simulink model "mvmama001_stltse004"  (R2021a)
settings: Solver=FixedStepAuto  StartTime=0.0  StopTime=500  RelTol=1e-3
undefined symbols (not defined in the file or in its folder): InputPWM, WheelSpeed
libraries: arduinolib x10, pid_lib x1, mobileRoboticsTrainingLib x1
settings Model: SILPILModeSetting=veronly  ExtModeTrigDuration=2  Creator=User  LastModifiedBy=Amandla Mvimbi
settings OptimizationCC: EnhancedBackFolding=on  PassReuseOutputArgsAs=Individual arguments  ZeroExternalMemoryAtStartup=off  ZeroInternalMemoryAtStartup=off  MaxStackSize=64  OptimizeBlockOrder=speed  DifferentSizesBufferReuse=on  EfficientTunableParamExpr=on
settings DebuggingCC: ParameterTunabilityLossMsg=error
settings HardwareCC: ProdBitPerInt=16  ProdBitPerPointer=16  ProdBitPerSizeT=16  ProdBitPerPtrDiffT=16  ProdLargestAtomicFloat=None  ProdWordSize=8  ProdHWDeviceType=Atmel->AVR  UseEmbeddedCoderFeatures=off  UseSimulinkCoderFeatures=off
settings SFSimCC: MATLABDynamicMemAlloc=off
settings RTWCC: SystemTargetFile=ert.tlc  HardwareBoard=Arduino Leonardo  TemplateMakefile=ert_default_tmf  Toolchain=Arduino AVR
settings CodeAppCC: ForceParamTrailComments=on  IgnoreCustomStorageClasses=off  OperatorAnnotations=on  SimulinkDataObjDesc=on  SFDataObjDesc=on  InsertBlockDesc=on
settings ERTTargetCC: SupportContinuousTime=on  SupportNonInlinedSFcns=on  SupportVariableSizeSignals=on  ExtModeTransport=5  ExtModeStaticAllocSize=250  ExtModeMexFile=ext_serial_win32_comm_leonardo

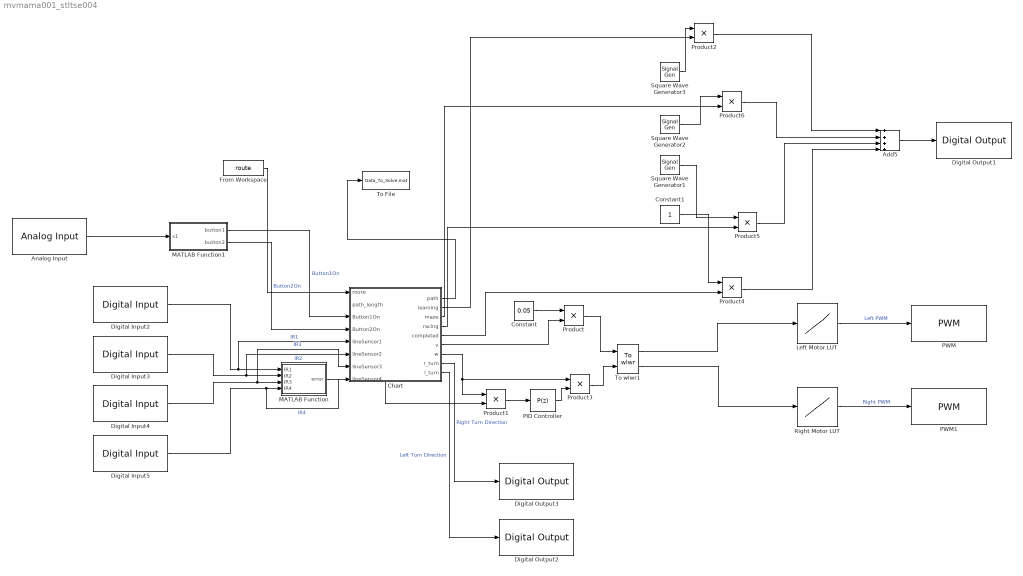
== system mvmama001_stltse004 ==
  Add5 : Sum  Inputs=++++
  Analog Input : arduinolib/Analog Input  pinNumber=0  ReadResultsOnly=off  ConversionTriggerSource=Software  ExternalTriggerType=uint32( 0 )  OutputDataType=uint16  EnableConversionCompleteNotify=off  EnableOuputStatus=off  SampleTime=-1  blockPlatform=arduino
  Chart : Stateflow chart  TreatAsAtomicUnit=on
      settings: PortSchema="{\"entries\":[{\"content\":{\"sides\":[{\"content\":{\"connectorIds\":[\"In7\",\"In8\",\"In1\",\"In2\",\"In3\",\"In5\",\"In4\",\"In6\"]},\"type\":\"ConnectorPlacement.EquallySpacedRectSide\",\"uuid\":\"badfc6b2-29c2-4b15-bfb9-62e4da121403\"},{\"content\":{\"connectorIds\":[\"Out9\",\"Out1\",\"Out3\",\"Out4\",\"Out2\",\"Out5\",\"Out6\",\"Out8\",\"Out7\"],\"side\":\"RIGHT\"},\"type\":\"ConnectorPlacement.EquallySpacedRectSide\",\"uuid\":\"19ffdcd3-74e5-47dc-b9d4-6ea0e9598c3b\"},{\"content\":{\"connectorIds\":[],\"side\":\"TOP\"},\"type\":\"ConnectorPlacement.EquallySpacedRectSide\",\"uuid\":\"4f1e845d-b34d-4676-ae53-c7ee998e6419\"}]},\"type\":\"ConnectorPlacement.EquallySpacedConnector\",\"uuid\":\"d87d8507-4bd7-4ce8-9c9b-ea7230bf73eb\"}],\"packageUris\":[\"http://schema.mathworks.com/mf0/Connector/R2020b\"],\"version\":\"1.0\"}"
  Constant : Constant  Value=0.05
  Constant1 : Constant
  Digital Input2 : arduinolib/Digital Input  pinNumber=8  mode=Default  Direction=input  SampleTime=0.1  blockPlatform=arduino
  Digital Input3 : arduinolib/Digital Input  pinNumber=9  mode=Default  Direction=input  SampleTime=0.1  blockPlatform=arduino
  Digital Input4 : arduinolib/Digital Input  pinNumber=10  mode=Default  Direction=input  SampleTime=0.1  blockPlatform=arduino
  Digital Input5 : arduinolib/Digital Input  pinNumber=11  mode=Default  Direction=input  SampleTime=0.1  blockPlatform=arduino
  Digital Output1 : arduinolib/Digital Output  pinNumber=13  Direction=output  blockPlatform=arduino
  Digital Output2 : arduinolib/Digital Output  pinNumber=4  Direction=output  blockPlatform=arduino
  Digital Output3 : arduinolib/Digital Output  pinNumber=7  Direction=output  blockPlatform=arduino
  From Workspace : FromWorkspace  VariableName=route
  Left Motor LUT : Lookup_n-D  NumberOfTableDimensions=1  BreakpointsForDimension1=WheelSpeed  Table=InputPWM  InterpMethod=Nearest  ExtrapMethod=Clip  InternalRulePriority=Speed  RndMeth=Simplest  InputSameDT=on
  MATLAB Function : MATLAB Function  TreatAsAtomicUnit=on
  MATLAB Function1 : MATLAB Function  TreatAsAtomicUnit=on
  PID Controller : pid_lib/PID Controller  Controller=P  Form=Parallel  TimeDomain=Discrete-time  UseExternalTs=off  SampleTime=-1  IntegratorMethod=Forward Euler  FilterMethod=Forward Euler  ControllerParametersSource=internal  P=0.6  I=0.8  D=1e-8  UseFilter=on  N=100  TunerSelectOption=Transfer Function Based (PID Tuner App)  InitialConditionSource=internal  InitialConditionForIntegrator=2  InitialConditionForFilter=0  DifferentiatorICPrevScaledInput=0  ExternalReset=none  TrackingMode=off  Kt=1  LimitOutput=off  SatLimitsSource=internal  UpperSaturationLimit=inf  LowerSaturationLimit=-inf  LinearizeAsGain=on  AntiWindupMode=none  Kb=1  POutMin=[]  POutMax=[]  IOutMin=[]  IOutMax=[]  DOutMin=[]  DOutMax=[]  NOutMin=[]  NOutMax=[]  SumOutMin=[]  SumOutMax=[]  SaturationOutMin=[]  SaturationOutMax=[]  PParamMin=[]  PParamMax=[]  IParamMin=[]  IParamMax=[]  DParamMin=[]  DParamMax=[]  NParamMin=[]  NParamMax=[]  KbParamMin=[]  KbParamMax=[]  KtParamMin=[]  KtParamMax=[]  KbOutMin=[]  KbOutMax=[]  KtOutMin=[]  KtOutMax=[]  IntegratorOutMin=[]  IntegratorOutMax=[]  FilterOutMin=[]  FilterOutMax=[]  SumI1OutMin=[]  SumI1OutMax=[]  SumI2OutMin=[]  SumI2OutMax=[]  SumI3OutMin=[]  SumI3OutMax=[]  SumI4OutMin=[]  SumI4OutMax=[]  SumDOutMin=[]  SumDOutMax=[]  DifferentiatorOutMin=[]  DifferentiatorOutMax=[]  FilterDiffOutCoefMin=[]  FilterDiffOutCoefMax=[]  ReciprocalOutMin=[]  ReciprocalOutMax=[]  SumDenOutMin=[]  SumDenOutMax=[]  SumNumOutMin=[]  SumNumOutMax=[]  DivideOutMin=[]  DivideOutMax=[]  UdiffTsProdOutMin=[]  UdiffTsProdOutMax=[]  NTsProdOutMin=[]  NTsProdOutMax=[]  UintegralTsProdOutMin=[]  UintegralTsProdOutMax=[]  UngainTsProdOutMin=[]  UngainTsProdOutMax=[]  IntegratorContinuousStateAttributes=''  IntegratorStateMustResolveToSignalObject=off  IntegratorRTWStateStorageClass=Auto  FilterContinuousStateAttributes=''  FilterStateMustResolveToSignalObject=off  FilterRTWStateStorageClass=Auto  ParallelPVariant=InternalParameters  IdealPVariant=Disabled  IVariant=Disabled  DVariant=Disabled  IntegratorVariant=Disabled  SatVariant=Disabled  AWVariant=Disabled  PCopyVariant=Disabled  TRVariant=Disabled  FdbkBlocksVariant=Forward  IdealPFdbkVariant=Disabled  SatFdbkVariant=Disabled  DerivativeFilterVariant=Disabled  NVariant=Disabled  NCopyVariant=Disabled_SignalSpec  FilterICVariant=Disabled  IntegratorICVariant=Disabled  ExternalResetVariant=Disabled  TRSumVariant=Passthrough  SumFdbkVariant=Disabled  SumVariant=Passthrough_P  TsampFilterVariant=InternalTs  TsampNgainVariant=Passthrough  TsampIntegralVariant=Disabled_SignalSpec  ExternalSaturationOutDataTypeStr=Inherit: Same as second input
  PWM : arduinolib/PWM  pinNumber=5  frequencyType=Default  desiredFrequency=490.2  achievableFrequency=490.2
  PWM1 : arduinolib/PWM  pinNumber=6  frequencyType=Default  desiredFrequency=490.2  achievableFrequency=490.2
  Product{,1..6} (7 alike) : Product
  Right Motor LUT : Lookup_n-D  NumberOfTableDimensions=1  BreakpointsForDimension1=WheelSpeed  Table=InputPWM  InterpMethod=Nearest  ExtrapMethod=Clip  InternalRulePriority=Speed  RndMeth=Simplest  InputSameDT=on
  Square Wave Generator1 : SignalGenerator  WaveForm=square  Frequency=5
  Square Wave Generator2 : SignalGenerator  WaveForm=square  Frequency=2
  Square Wave Generator3 : SignalGenerator  WaveForm=square
  To File : ToFile  Filename=Data_To_Solve.mat  MatrixName=path_raw  SampleTime=5
  To wlwr1 : mobileRoboticsTrainingLib/To wlwr  axleLength=axleLength  wheelR=wheelR
  wires:
  Product1/1 -> PID Controller/1
  MATLAB Function/1(error) -> Product1/2
  Product/1 -> To wlwr1/1
  Right Motor LUT/1 -> PWM1/1  "Right PWM"
  Square Wave Generator1/1 -> Product5/1
  Add5/1 -> Digital Output1/1
  Chart/4(racing) -> Product5/2
  Chart/2(completed) -> Product4/2
  Square Wave Generator2/1 -> Product6/1
  Constant/1 -> Product/1
  MATLAB Function1/1(button1) -> Chart/1(Button1On)  "Button1On"
  Product4/1 -> Add5/4
  Product6/1 -> Add5/2
  Constant1/1 -> Product4/1
  Product5/1 -> Add5/3
  Digital Input3/1 -> Chart/5(lineSensor2), MATLAB Function/2(IR2)  "IR2"
  Digital Input2/1 -> Chart/3(lineSensor1), MATLAB Function/1(IR1)  "IR1"
  Chart/3(maze) -> Product6/2
  Chart/6(w) -> Product1/1, Product3/1
  Digital Input4/1 -> Chart/4(lineSensor3), MATLAB Function/3(IR3)  "IR3"
  Analog Input/1 -> MATLAB Function1/1(s1)
  Left Motor LUT/1 -> PWM/1  "Left PWM"
  Digital Input5/1 -> Chart/6(lineSensor4), MATLAB Function/4(IR4)  "IR4"
  Product3/1 -> To wlwr1/2
  Chart/8(r_turn) -> Digital Output3/1  "Right Turn Direction"
  Square Wave Generator3/1 -> Product2/1
  Product2/1 -> Add5/1
  Chart/1(learning) -> Product2/2
  MATLAB Function1/2(button2) -> Chart/2(Button2On)  "Button2On"
  Chart/5(v) -> Product/2
  PID Controller/1 -> Product3/2
  To wlwr1/2 -> Right Motor LUT/1
  To wlwr1/1 -> Left Motor LUT/1
  Chart/7(l_turn) -> Digital Output2/1  "Left Turn Direction"
  Chart/9(path) -> To File/1
  From Workspace/1 -> Chart/7(route)

== matlab function mvmama001_stltse004/MATLAB Function1 ==
  data: s1 input; button1 output; button2 output
function [button1, button2] = fcn(s1)
p1 = 0;
p2 = 0;
if s1 <= 100
    p1 = 1;
end
if s1 > 100 && s1 < 200
    p2 = 1;
end
button1 = p1;
button2 = p2;

== matlab function mvmama001_stltse004/MATLAB Function ==
  data: IR1 input; error output; IR2 input; IR3 input; IR4 input
function error = fcn(IR1, IR2, IR3, IR4)
% Sets the number of sensors on the line to 0
numberof0 = 0;
% Checks if IR2 is on the line
if IR2 == 0 
    % Increments the count of number of sensors on the line
    numberof0 = numberof0 + 1; 
end
% Checks if IR3 is on the line
if IR3 == 0 
    % Increments the count of number of sensors on the line
    numberof0 = numberof0 + 1; 
end
% If neither of the two middle sensors are on the line, stop the robot
if numberof0 == 0 
    CurrentDeveation = 0;
else
    % This formula determines the currevnt deviation of the robot
    CurrentDeveation = ((IR2*2)+(IR3*-2))/numberof0;
end
% Calculates the error from the current deviation
error = 0 - CurrentDeveation;

== stateflow chart mvmama001_stltse004/Chart ==
  state RightT1
    entry:
    v=1;
    w=1;
    r_turn=-1;
    l_turn =-1;
    length1=length1+1;
  state Button1_On
    entry:
    learning =1;
    v=-1;
    w=-1;
    r_turn=-1;
    l_turn=-1;
    length1=1;
    path = zeros(1,100);
  state Start
    entry:
    completed = 0;
    maze=0;
    learning =0;
    racing =0;
    v=0;
    w=0;
    r_turn=-1;
    l_turn=-1;
    length1=0;
    path = zeros(1,100);
  state Junction_Detect
    entry:
    v=1;
    length1=length1+1;
  state Forward
    entry:
    v=1;
  state Button2_On
    entry:
    direction= 0;
    v=-1;
    w=-1;
    r_turn=-1;
    l_turn=-1;
    length1= 2;
    maze= 0;
    racing =1;
  state Right
    entry:
    v=0;
  state Junction_Detect1
    entry:
    v=1;
    direction = route(path_length+1);
  state Forward1
    entry:
    v=1;
  state Right1
    entry:
    v=0;
  state Left
    entry:
    v=0;
  state Straight
    entry:
    v=1;
  state Cross
  state Left1
    entry:
    v=0;
  state Straight1
    entry:
    v=1;
  state Right_Detect
    entry:
    v=1;
    w=0;
    r_turn=1;
    l_turn =-1;
  state Cross1
  state Backward
    entry:
    v=1;
    w=1;
    r_turn=-1;
    l_turn =-1;
    path(length1)=2;
  state Check
    entry:
    v=-0.5;
  state Check2
  state Right_Detect1
    entry:
    v=1;
    w=0;
    r_turn=1;
    l_turn =-1;
  state Straight_Detect
    entry:
    v=0;
  state Left_Detect
    entry:
    v=1;
    w=0;
    r_turn=-1;
    l_turn =1;
  state Check3
    entry:
    v=-0.5;
  state Check4
  state Stop1
    entry:
    completed=1;
    racing =1;
    v=0;
    w=0;
    r_turn=-1;
    l_turn =-1;
  state Straight_Detect1
    entry:
    l_turn=1;
    r_turn =-1;
    v=1;
  state Left_Detect1
    entry:
    v=1;
    w=0;
    r_turn=-1;
    l_turn =1;
  state RightTurn
    entry:
    v=1;
    w=0;
    r_turn=1;
    l_turn =-1;
  state RightT
    entry:
    v=1;
    w=1;
    r_turn=-1;
    l_turn =-1;
    path(length1)=4;
  state Continue
    entry:
    v=1;
    w=1;
    r_turn=-1;
    l_turn =-1;
    path(length1)=3;
  state RightTurn1
    entry:
    v=1;
    w=0;
    r_turn=1;
    l_turn =-1;
  state LeftT
    entry:
    v=0;
    w=1;
    r_turn=-1;
    l_turn =-1;
    path(length1)=1;
  state Continue1
    entry:
    v=1;
    w=1;
    r_turn=-1;
    l_turn =-1;
    length1=length1+1;
  state LeftTurn
    entry:
    v=1;
    w=0;
    r_turn=-1;
    l_turn =1;
  state LeftT1
    entry:
    v=0;
    w=1;
    r_turn=-1;
    l_turn =-1;
    length1=length1+1;
  state LeftTurn1
    entry:
    v=1;
    w=0;
    r_turn=-1;
    l_turn =1;
  state DeadEnd
    entry:
    v=1;
    w=0;
    r_turn=-1;
    l_turn =1;
  state DeadEnd1
    entry:
    v=1;
    w=0;
    r_turn=-1;
    l_turn =1;
  state TurnAround
    entry:
    v=1;
    w=0;
    r_turn=-1;
    l_turn =1;
  state Backward1
    entry:
    v=1;
    w=1;
    r_turn=-1;
    l_turn =-1;
    path(length1)=2;
  state TurnAround1
    entry:
    v=1;
    w=0;
    r_turn=-1;
    l_turn =1;
  state Stop
    entry:
    learning =0;
    maze =1;
    v=0;
    w=0;
    r_turn=-1;
    l_turn =-1;
  state crossVerification
    entry:
    v = 1;
  RightT -> Forward
  Continue -> Forward
  RightT1 -> Forward1
  Continue1 -> Forward1
  (default) -> Start
  RightTurn1 -> RightT1 : [lineSensor2==0&&lineSensor3==0]
  Button1_On -> Forward
  Forward -> Junction_Detect : [lineSensor1 == 0 || lineSensor2 == 1&& lineSensor3 == 1|| lineSensor4 == 0 ]
  Junction_Detect -> Right [order 1] : [lineSensor4 ==0&&lineSensor1~=0]
  Backward -> Forward
  Start -> Button1_On : [Button1On==1]
  LeftT -> Forward
  Right -> Continue [order 2] : after(1,sec)
  Junction_Detect -> Left [order 3] : [lineSensor1==0]
  Junction_Detect -> Straight [order 2] : after(0.6,sec)[lineSensor2==1&&lineSensor3==1]
  Button2_On -> Forward1
  Forward1 -> Junction_Detect1 : [lineSensor1 == 0 || lineSensor2 == 1&& lineSensor3 == 1|| lineSensor4 == 0 ]
  Junction_Detect1 -> Right1 [order 1] : [direction ==4]
  Right -> Right_Detect [order 1] : [lineSensor4 ==0 && lineSensor2 ==1&& lineSensor3==1]
  Backward1 -> Forward1
  LeftT1 -> Forward1
  Junction_Detect1 -> Left1 [order 3] : [direction==1]
  Junction_Detect1 -> Straight1 [order 2] : [direction ==3]
  Junction_Detect1 -> Stop1 [order 4] : [direction ==0]
  Right1 -> Continue1 [order 1] : after(1,sec)
  Right1 -> Right_Detect1 [order 2] : [lineSensor4 ==0 && lineSensor2 ==1&& lineSensor3==1]
  Stop -> Button2_On : [Button2On == 1]
  Left -> Cross [order 2] : [lineSensor1==0&&lineSensor2==0&&lineSensor3==0&&lineSensor4==0]
  Left -> Check [order 1] : [lineSensor1==0&&lineSensor2==1&&lineSensor3==1]
  Cross -> Check2 : after(1,sec)
  Left -> Left_Detect [order 3] : after(1,sec)
  Straight -> Straight_Detect : after(0.2,sec)
  Left1 -> Cross1 [order 2] : [lineSensor1==0&&lineSensor2==0&&lineSensor3==0&&lineSensor4==0]
  Left1 -> Check3 [order 1] : [lineSensor1==0&&lineSensor2==1&&lineSensor3==1]
  Cross1 -> Check4 : after(1,sec)
  Left1 -> Left_Detect1 [order 3] : after(1,sec)
  Straight1 -> Straight_Detect1 : after(0.2,sec)
  Right_Detect -> RightTurn : after(1,sec)
  Check -> Left_Detect : after(1,sec)
  Check2 -> crossVerification [order 1] : [lineSensor1 == 0 && lineSensor2 == 0&& lineSensor3 == 0 && lineSensor4 == 0]
  Check2 -> Left_Detect [order 2]
  Straight_Detect -> Continue [order 2]
  Right_Detect1 -> RightTurn1 : after(1,sec)
  Check3 -> Left_Detect1 : after(0.2,sec)
  Check4 -> Left_Detect1
  Straight_Detect -> DeadEnd [order 1] : [lineSensor1 == 1 && lineSensor2 == 1&& lineSensor3 == 1 && lineSensor4 == 1]
  crossVerification -> Left_Detect [order 1] : after(1,sec)[lineSensor1 ~= 0 || lineSensor2 ~= 0|| lineSensor3 ~= 0 || lineSensor4 ~= 0]
  Left_Detect -> LeftTurn : after(1.5,sec)
  TurnAround -> Backward : [lineSensor2==0&&lineSensor3==0]
  Straight_Detect1 -> Continue1 [order 2]
  RightTurn -> RightT : [lineSensor2==0&&lineSensor3==0]
  Straight_Detect1 -> DeadEnd1 [order 1] : [lineSensor1 == 1 && lineSensor2 == 1&& lineSensor3 == 1 && lineSensor4 == 1]
  Left_Detect1 -> LeftTurn1 : after(1.5,sec)
  LeftTurn -> LeftT : [lineSensor2==0&&lineSensor3==0]
  LeftTurn1 -> LeftT1 : [lineSensor2==0&&lineSensor3==0]
  DeadEnd -> TurnAround : after(1.5,sec)
  DeadEnd1 -> TurnAround1 : after(1.5,sec)
  TurnAround1 -> Backward1 : [lineSensor2==0&&lineSensor3==0]
  crossVerification -> Stop [order 2] : after(2,sec)[lineSensor1 == 0 && lineSensor2 == 0&&lineSensor3 == 0 &&  lineSensor4 == 0]
  data: learning output; completed output; maze output; racing output; v output; Button1On input; Button2On input; lineSensor1 input; lineSensor3 input; lineSensor2 input; lineSensor4 input; w output; l_turn output; r_turn output; path output; route input; direction local; length1 local; path_length input
